simulink model "test_Eq_euler"  (R2018a)
settings: Solver=VariableStepAuto  StartTime=0.0  StopTime=10.0  RelTol=1e-3
settings Model: Creator=LabT5  LastModifiedBy=LabT5

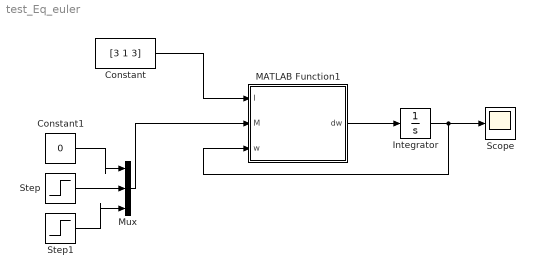
== system test_Eq_euler ==
  Constant : Constant  Value=[3 1 3]
  Constant1 : Constant  Value=0
  Integrator : Integrator  InitialCondition=[0 0 0]
  MATLAB Function1 : MATLAB Function  TreatAsAtomicUnit=on
  Mux : Mux  Inputs=3
  Scope : Scope
  Step : Step  After=-1  SampleTime=0
  Step1 : Step  After=-1  SampleTime=0
  wires:
  MATLAB Function1/1(dw) -> Integrator/1
  Constant/1 -> MATLAB Function1/1(I)
  Integrator/1 -> MATLAB Function1/3(w), Scope/1
  Mux/1 -> MATLAB Function1/2(M)
  Constant1/1 -> Mux/1
  Step/1 -> Mux/2
  Step1/1 -> Mux/3

== matlab function test_Eq_euler/MATLAB Function1 ==
  data: I input; dw output; M input; w input
function dw = Eq_Euler(I,M,w)
wx = w(1);
wy = w(2);
wz = w(3);
Ix = I(1);
Iy = I(2);
Iz = I(3);

Mx = M(1);
My = M(2);
Mz = M(3);

dwx = (Mx - wy*wz*(Iz - Iy))/Ix;
dwy = (My - wx*wz*(Ix - Iz))/Iy;
dwz = (Mz - wx*wy*(Iy - Ix))/Iz;

dw=[dwx dwy dwz]';
